simulink model "model"  (R2020b)
settings: Solver=VariableStepAuto  StartTime=0.0  StopTime=10  FixedStep=0.0001  RelTol=1e-8  AbsTol=1e-8
PostLoadFcn:
  | path = fileparts(which(bdroot))
  | cd(path)
  | masscgI = xlsread('mass,cg,I','mass,cg,I');
  | ThrustTable = xlsread('F15_Thrust','Sheet1');
  | u = xlsread('../../scp_new_problem/src/u.csv','u');
  | moments = xlsread('../../scp_new_problem/src/moments.csv','moments');
  | x = xlsread('../../scp_new_problem/src/x.csv','x');
  | ignition_time = u(3, 1)
InitFcn:
  | HeightAboveSeaLevel = 5.4419142084;
  | 
  | GustStart = 1;
  | GustLength = [120, 130, 80];
  | GuestAmplitude = [ 2.5, -2.5,  1];
  | 
  | ShearSpeed = 4;
  | ShearDirection = 75;
  | 
  | Croll = 0.001 * (rand - 0.5);
  | Cyaw = 0.05 * (rand - 0.5);
  | Cside = 0.001 * (rand - 0.5);
  | 
  | GustStart = 2 * rand;
  | GustLength = [100 + 50 * (rand - 0.5), 100 + 50 * (rand - 0.5), 100 + 50 * (rand - 0.5)];
  | GuestAmplitude = [ 5 * (rand - 0.5), 5 * (rand - 0.5),  5 * (rand - 0.5)];
  | 
  | ShearSpeed = 5 * rand;
  | ShearDirection = 360 * rand;
  | 
  | HeightAboveSeaLevel = rand * 1000;
values from neighbouring files (symbols this model uses):
  D = zeros(size(B))    [RocketOutputFunction.m]    (also in StateSpaceController.m; TimeDelayCompensationElevator.m = [0; 0])
  F = eye(6)    [MEKFAttitudeOnly.m]
  K = 1.1    [DATCOMvsOR.m]    (also in Forces_and_Moments_Calculator.m; MEKF.m = (P * H.') / (H * P * H.' + V); MEKFAttitudeOnly.m = P2 * H' * inv(S); MEKF_old.m = (P * H.') / (H * P * H.' + V))
  q = x(13:16)    [AdaptiveLQR.m]    (also in MEKF.m = nominal_state(4:7); MEKFAttitudeOnly.m = [1 0 0 0]; MEKF_old.m = nominal_state(4:7); NonlinearStateEstimationForActuatorDelay.m = x(4:7))
  r = [0; 0; -(rocket_length - Average_cg)]    [StateSpaceController.m]    (also in TimeDelayCompensationElevator.m = [0;0]; Tracker.m)
  s = linspace(0, 100, nums)    [ImpactVelocityFunction.m]    (also in ImpactVelocityNotParallelMatlab.m = 1:5:500; ParallelImpactVelocity.m = .1:.01:500; ParralelRun.m = linspace(5,7, nums); RunImpactVelocityParforCompiled.m = 1:0.1:500)
  whentoignite = [s(row); v(col)]    [SecondPartLandingAlgorithm.m]
undefined symbols (not defined in the file or in its folder): Angle, Axis, deg, e0_0, e1_0, e2_0, e3_0, Earth, Kri, Light, magnitude, MIL, rad, WGS84
libraries: vrlib x8, shared6dof x8, aerolibutil x7, aerolibconvert2 x6, simulink x6, aerolibasang x4, sharedtransform x4, aerolibwind2 x3, pid_lib x3, sharedschedule x2, robotcorelib x2, sharedutil x2
(part 4 of 4)

== matlab function model/Subsystem/Acceleration Calculator1/Forces And Moments simple model ==
  settings: updateMethod=DISCRETE
  data: Mach input; Airspeed input size=[3 1]; AoA input; Density input; Temperature input; DynamicPressure input; CenterOfMassX input; Thrust input; Forces output; body_angular_velocity input; Roll_Torque input; Xe input; Moments output; Weight input; CFrictionDrag output
function [Forces, Moments, CFrictionDrag]  = forces(Mach, Airspeed, AoA, Density, Temperature, DynamicPressure, CenterOfMassX, Thrust, body_angular_velocity, Roll_Torque, Xe, Weight)
    persistent ThetaRotation
    if isempty(ThetaRotation)
         ThetaRotation = eye(3);
    end
    
    persistent Croll_p
    if isempty(Croll_p)
        Croll_p = 0.03 * (rand - 0.5);
    end
    %% Rocket Shape Constants
    Reference_Diameter = 7.62e-2;
    Reference_Radius = Reference_Diameter / 2;
    Reference_Area = Reference_Radius^2 * pi;
    
    NoseCone_Length = 15e-2;
    BodyTube_Length = 80e-2; 
    NoseCone_WetArea = pi * Reference_Radius * NoseCone_Length;          % pi*r*l 
    BodyTube_WetArea = pi * Reference_Radius * 2 * BodyTube_Length;      % pi*d*l
    NoseCone_PlanformArea = Reference_Diameter * NoseCone_Length / 2;
    BodyTube_PlanformArea = Reference_Diameter * BodyTube_Length;
    
    SurfaceRoughness = 20e-6;
    
    sinphi = Reference_Radius / hypot(Reference_Radius, NoseCone_Length);
    BodyTube_CP = 0.55;
    NoseCone_CP = 0.1;
    PitchCenterX = 0;
   
    
    COT_to_COM = .95 - CenterOfMassX; %get actual value and change over time as solid motor burns
    
    %% General Constants
    K = 1.1;
   
    %% Coefficients
    angularrate_local = ThetaRotation \ body_angular_velocity;
    [CN, Cpitch] = CalculatePitchAndNormalCDs(Mach, K, Reference_Diameter, AoA, Airspeed, angularrate_local(2), NoseCone_Length, BodyTube_Length, Reference_Area, CenterOfMassX, PitchCenterX, NoseCone_PlanformArea, BodyTube_PlanformArea, NoseCone_CP, BodyTube_CP);

    Cbase = .12 + .13*Mach^2;
    CFrictionDrag = CalculateFrictionDrag(Temperature, Density, Reference_Radius, Reference_Area, SurfaceRoughness, NoseCone_Length, BodyTube_Length, Airspeed, Mach, NoseCone_WetArea, BodyTube_WetArea);
    Cpressure = PressureDragForce(sinphi);
    
    Cdrag = Cbase + CFrictionDrag + Cpressure;
    Caxial = AxialDragMul(AoA) * Cdrag;

    Cyaw = 0;
    Cside = 0;
    Croll = 0;
    
     %% Random Noise to pitch and yaw coefficients in the range of +- 5e-4
    %Cpitch = Cpitch + .1 * (rand - 0.5);
    %Cyaw = Cyaw + .1 * (rand - 0.5);
    %Croll = Croll_p + .0001 * (rand - 0.5);
    %% Forces and Moments
    lengtha = norm(Airspeed(1:2));
    
    cosa = Airspeed(1) / lengtha;
    sina = Airspeed(2) / lengtha;

    ThetaRotation = [cosa, -sina, 0; sina, cosa, 0; 0, 0, 1];
    
    z = DynamicPressure * Reference_Area;
    Thrust_moment = COT_to_COM * [Thrust(1:2); 0] + [0;0; Roll_Torque];
    
    Forces = ThetaRotation * z * -[CN; Cside; Caxial] + Thrust - Weight;
    Moments = ThetaRotation * (z * Reference_Diameter * [-Cyaw; Cpitch; Croll]) + Thrust_moment;
    
    if Xe(3) <= 0
        Forces = [0;0; dot(Forces, [0,0,1])];
        Moments = [0; 0; 0];
    end
    
end

== matlab function model/Subsystem4/Desired Quaternion ==
  settings: updateMethod=DISCRETE
  data: current_direction input; Desired_Direction input; Error_Quaternion output size=[1 4]
function Error_Quaternion  = func(current_direction, Desired_Direction)
    w = cross(current_direction, Desired_Direction);
    q = [dot(current_direction, Desired_Direction),w]; 
    Error_Quaternion = normalize([q(1) + norm(q), q(2:4)]);

== matlab function model/Subsystem/Acceleration Calculator1/Subsystem/AngleOfAtack1 ==
  settings: updateMethod=DISCRETE
  data: Airspeed input; AoA output
function AoA = AngleOfAttack(Airspeed)
    AoA = acos(Airspeed(3) / norm(Airspeed));
        
    if norm(Airspeed) <= .01
        AoA = 0;
    end
end

== matlab function model/Subsystem4/Desired Quaternion1 ==
  settings: updateMethod=DISCRETE
  data: Desired_Direction input; a output size=[1 4]
function a  = func(Desired_Direction)
    m = sqrt(2 + 2 * Desired_Direction(3));
    w = (1 / m) * [-Desired_Direction(2) Desired_Direction(1) 0];
    a =  [0.5 * m, w];

== matlab function model/Control/Affine LQR (New LQR at every x seconds)/MATLAB Function1 ==
  settings: updateMethod=DISCRETE
  data: state input; u input; K_x_out output; time input; k_0_out output
function [K_x_out, k_0_out] = fcn(state, u, time)
  coder.extrinsic('affine_controller'); 
  persistent last_time K_x k_0

  if isempty(last_time)
    last_time = 0;
    K_x = zeros(3, 9);
    k_0 = zeros(3, 1);
%     [K_x, k_0, t, ~] = affine_controller(state, u, 3.45 - time);
    [K_x, k_0, ~] = affine_controller(state, u, inf);
  end
  
  if time - last_time > 10
%     [K_x, k_0, t, ~] = affine_controller(state, u, 3.45 - time);
    [K_x, k_0, ~] = affine_controller(state, u, inf);
  end
  
%   [ ~, ix ] = min( abs( t - (time - last_time) ) );
%   
%   K_x_out = K_x(:, :, ix);
%   k_0_out = k_0(:, :, ix);
  K_x_out = K_x;
  k_0_out = k_0;
  
  last_time = time;
end

== matlab function model/MATLAB Function2 ==
  data: Inertia input; state input; u input; estimated_state output; ThrustTable input; time input; masscgI input
function estimated_state = fcn(Inertia, state, u, ThrustTable, time, masscgI)
  coder.extrinsic('NonlinearStateEstimationForActuatorDelay'); 
  estimated_state = zeros(15, 1);
  estimated_state = NonlinearStateEstimationForActuatorDelay(Inertia, state, u, ThrustTable, time, 0, masscgI);
end

== matlab function model/MATLAB Function3 ==
  data: time input; final_state output; state input
function final_state = fcn(time, state)
  coder.extrinsic('RunNonlinearStateEstimationForActuatorDelay')
  final_state = zeros(16, 1);
  Moments_t = [0 3.45]';
  Moments_data = [0 0 0; 0 0 0];
  Moments = [Moments_t Moments_data];
  final_state = RunNonlinearStateEstimationForActuatorDelay(time, state, Moments);
end

== matlab function model/Thrust Magnitude (N)/MATLAB Function ==
  settings: updateMethod=DISCRETE
  data: whentoignite input; incoastingphase input; y output; state input
function y = fcn(whentoignite, incoastingphase, state)
    persistent burnstarted
    if isempty(burnstarted)
        burnstarted = 0;
    end
    
    tol = 5e-2;
    if sum(sum(abs(bsxfun(@minus, whentoignite, state)), 1) < tol) > 0 && incoastingphase % take the absolute of subtracted matrix and sum columwise, find number of elements less than tol, if greater than 0 ignite
        burnstarted = 1;
    end
     
    y = burnstarted;

== matlab function model/Moment to Force and Actuator Model/50Hz delay ==
  settings: updateMethod=DISCRETE
  data: time input; input input; delayed_input output
function delayed_input = Servo(time, input)
    persistent lastupdate
    if isempty(lastupdate)
        lastupdate = [0;0;0];
    end
    
    servo_frequency = 50; %Hz
    if mod(time, 1/servo_frequency) == 0
        lastupdate = input;
    end    
        
    delayed_input = lastupdate;
end

== matlab function model/Subsystem/Acceleration Calculator/Subsystem/AngleOfAtack1 ==
  settings: updateMethod=DISCRETE
  data: Airspeed input; AoA output
function AoA = AngleOfAttack(Airspeed)
    AoA = acos(Airspeed(3) / norm(Airspeed));
        
    if norm(Airspeed) <= .01
        AoA = 0;
    end
end

== matlab function model/Subsystem/Acceleration Calculator/Forces And Moments simple model ==
  settings: updateMethod=DISCRETE
  data: Mach input; Airspeed input size=[3 1]; AoA input; Density input; Temperature input; DynamicPressure input; CenterOfMassX input; Thrust input; Forces output; body_angular_velocity input; Roll_Torque input; Xe input; Moments output; Weight input; CFrictionDrag output
function [Forces, Moments, CFrictionDrag]  = forces(Mach, Airspeed, AoA, Density, Temperature, DynamicPressure, CenterOfMassX, Thrust, body_angular_velocity, Roll_Torque, Xe, Weight)
    persistent ThetaRotation
    if isempty(ThetaRotation)
         ThetaRotation = eye(3);
    end
    
    persistent Croll_p
    if isempty(Croll_p)
        Croll_p = 0.03 * (rand - 0.5);
    end
    %% Rocket Shape Constants
    Reference_Diameter = 7.62e-2;
    Reference_Radius = Reference_Diameter / 2;
    Reference_Area = Reference_Radius^2 * pi;
    
    NoseCone_Length = 15e-2;
    BodyTube_Length = 80e-2; 
    NoseCone_WetArea = pi * Reference_Radius * NoseCone_Length;          % pi*r*l 
    BodyTube_WetArea = pi * Reference_Radius * 2 * BodyTube_Length;      % pi*d*l
    NoseCone_PlanformArea = Reference_Diameter * NoseCone_Length / 2;
    BodyTube_PlanformArea = Reference_Diameter * BodyTube_Length;
    
    SurfaceRoughness = 20e-6;
    
    sinphi = Reference_Radius / hypot(Reference_Radius, NoseCone_Length);
    BodyTube_CP = 0.55;
    NoseCone_CP = 0.1;
    PitchCenterX = 0;
   
    
    COT_to_COM = .95 - CenterOfMassX; %get actual value and change over time as solid motor burns
    
    %% General Constants
    K = 1.1;
   
    %% Coefficients
    angularrate_local = ThetaRotation \ body_angular_velocity;
    [CN, Cpitch] = CalculatePitchAndNormalCDs(Mach, K, Reference_Diameter, AoA, Airspeed, angularrate_local(2), NoseCone_Length, BodyTube_Length, Reference_Area, CenterOfMassX, PitchCenterX, NoseCone_PlanformArea, BodyTube_PlanformArea, NoseCone_CP, BodyTube_CP);

    Cbase = .12 + .13*Mach^2;
    CFrictionDrag = CalculateFrictionDrag(Temperature, Density, Reference_Radius, Reference_Area, SurfaceRoughness, NoseCone_Length, BodyTube_Length, Airspeed, Mach, NoseCone_WetArea, BodyTube_WetArea);
    Cpressure = PressureDragForce(sinphi);
    
    Cdrag = Cbase + CFrictionDrag + Cpressure;
    Caxial = AxialDragMul(AoA) * Cdrag;

    Cyaw = 0;
    Cside = 0;
    Croll = 0;
    
     %% Random Noise to pitch and yaw coefficients in the range of +- 5e-4
    %Cpitch = Cpitch + .1 * (rand - 0.5);
    %Cyaw = Cyaw + .1 * (rand - 0.5);
    %Croll = Croll_p + .0001 * (rand - 0.5);
    %% Forces and Moments
    lengtha = norm(Airspeed(1:2));
    
    cosa = Airspeed(1) / lengtha;
    sina = Airspeed(2) / lengtha;

    ThetaRotation = [cosa, -sina, 0; sina, cosa, 0; 0, 0, 1];
    
    z = DynamicPressure * Reference_Area;
    Thrust_moment = COT_to_COM * [Thrust(1:2); 0] + [0;0; Roll_Torque];
    
    Forces = ThetaRotation * z * -[CN; Cside; Caxial] + Thrust - Weight;
    Moments = ThetaRotation * (z * Reference_Diameter * [-Cyaw; Cpitch; Croll]) + Thrust_moment;
    
    if Xe(3) <= 0
        Forces = [0;0; dot(Forces, [0,0,1])];
        Moments = [0; 0; 0];
    end
    
end

== matlab function model/Subsystem3/Subsystem2/Desired Quaternion ==
  settings: updateMethod=DISCRETE
  data: input_acceleration input; thrust_acceleration input; desired_quaternion output size=[1 4]; ln_quat output
function [desired_quaternion, ln_quat] = func(input_acceleration, thrust_acceleration)

    max_horizontal_acceleration = sin(deg2rad(10)) * thrust_acceleration;
    if norm(input_acceleration) > max_horizontal_acceleration
        input_acceleration = input_acceleration * max_horizontal_acceleration / norm(input_acceleration);
    end
    
    global_thrust = [input_acceleration.', (thrust_acceleration^2 - norm(input_acceleration)^2)^.5];
    
    if norm(global_thrust) == 0
        global_thrust = [0,0,1];
    end
    
    desired_quaternion = quatnormalize([ global_thrust(3) + norm(global_thrust), cross([0;0;1], global_thrust) ]);
%     test = quatnormalize([norm(global_thrust) + global_thrust(3), cross([0 0 1], global_thrust)]);
    
    if norm(desired_quaternion(2:4)) == 0
        ln_quat = [0 0 0];
    else
        ln_quat = desired_quaternion(2:4)/norm(desired_quaternion(2:4)) * desired_quaternion(1);
    end
    
%     desired_quaternion = [cos(pi/8) sin(pi/8) * [1 0 0]];
